simulink model "Aerotherme"  (R2019a)
settings: Solver=ode8  StartTime=0.0  StopTime=inf  FixedStep=0.1  RelTol=1e-3  EnableMultiTasking=on
values from neighbouring files (symbols this model uses):
  CorInt = tf(1 , [1 0])    [TP6.m]
  CorPD = tf([Td 1] , 1)*Kp    [TP6.m]
libraries: raspberrypilib x2, cstblocks x1
settings Model: SimulationMode=external  Creator=dorleans  LastModifiedBy=fereka231
settings SolverCC: PositivePriorityOrder=on
settings DataIOCC: ReturnWorkspaceOutputs=off
settings OptimizationCC: PassReuseOutputArgsAs=Individual arguments  MaxStackSize=64
settings DebuggingCC: ParameterPrecisionLossMsg=none  ParameterTunabilityLossMsg=error  SFUnexpectedBacktrackingDiag=warning  SFNoUnconditionalDefaultTransitionDiag=warning  ArithmeticOperatorsInVariantConditions=warning
settings HardwareCC: ProdBitPerPointer=32  ProdBitPerSizeT=32  ProdBitPerPtrDiffT=32  ProdLargestAtomicInteger=Long  ProdLargestAtomicFloat=Double  ProdWordSize=32  ProdHWDeviceType=ARM Compatible->ARM Cortex
settings ModelReferenceCC: PropagateSignalLabelsOutOfModel=off
settings SFSimCC: SimUseLocalCustomCode=off  MATLABDynamicMemAlloc=off
settings RTWCC: SystemTargetFile=ert.tlc  HardwareBoard=Raspberry Pi  TLCOptions="-aInlineSetEventsForThisBaseRateFcn=TLC_FALSE -aSuppressMultiTaskScheduler=TLC_FALSE  -aRateBasedStepFcn=0"  TemplateMakefile=ert_default_tmf  GenerateReport=on  RTWUseLocalCustomCode=off  Toolchain=GNU GCC Raspberry Pi  IncludeHyperlinkInReport=on  LaunchReport=on  GenerateTraceInfo=on  GenerateTraceReport=on  GenerateTraceReportSl=on  GenerateTraceReportSf=on  GenerateTraceReportEml=on
settings CodeAppCC: ForceParamTrailComments=on  IgnoreCustomStorageClasses=off  OperatorAnnotations=on  SimulinkDataObjDesc=on  SFDataObjDesc=on  MATLABFcnDesc=on  InsertBlockDesc=on  StateflowObjectComments=on  MATLABSourceComments=on
settings ERTTargetCC: SupportContinuousTime=on  SupportVariableSizeSignals=on

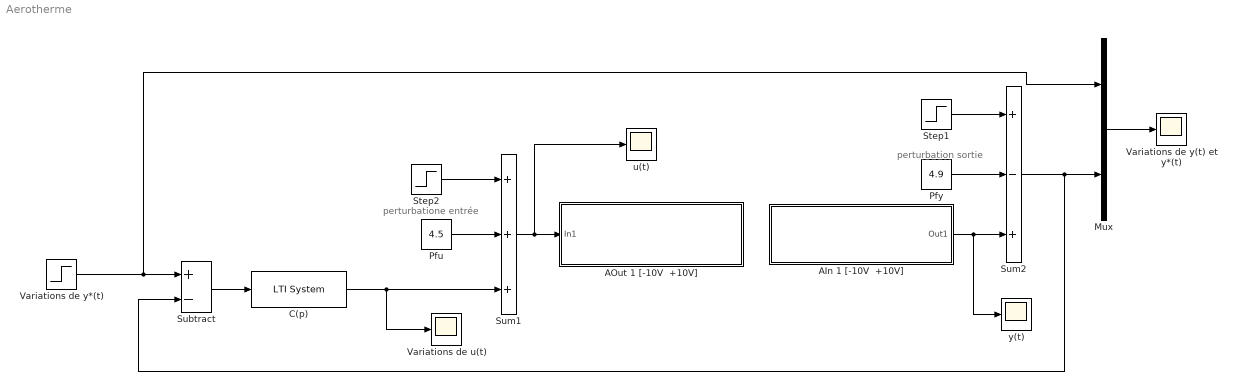
== system Aerotherme ==
  note: perturbatione entrée
  note: perturbation sortie
  AIn 1 [-10V  +10V] : Subsystem
      settings: OpenFcn=errordlg('Réalisé par Ph. Dorléans, H. Fleury','ESIX - UCBN')
      mask Display:
      | color('white');
      | plot([100,100,100,100],[100,100,100,100]);
      | plot([0,0,0,0],[0,0,0,0]);
      | color('blue');
      | text(99, 92, 'RASPBERRYPI', 'horizontalAlignment', 'right');
      | color('black');
      | text(50,60,'\fontsize{12}\bfAcquisition voie 1','texmode','on','horizontalAlignment','center','verticalAlignment','middle');
      | text(50,40,'\fontsize{10}\bfSPI Bus','texmode','on','horizontalAlignment','center','verticalAlignment','middle');
      | text(50,15,'Master Receiver SPI0 CE0' ,'horizontalAlignment', 'center');
  AOut 1 [-10V  +10V] : Subsystem
      settings: OpenFcn=errordlg('Réalisé par Ph. Dorléans, H. Fleury','ESIX - UCBN')
      mask Display:
      | color('white');
      | plot([100,100,100,100],[100,100,100,100]);
      | plot([0,0,0,0],[0,0,0,0]);
      | color('blue');
      | text(99, 92, 'RASPBERRYPI', 'horizontalAlignment', 'right');
      | color('black');
      | text(50,60,'\fontsize{12}\bfSortie analogique voie 1','texmode','on','horizontalAlignment','center','verticalAlignment','middle');
      | text(50,40,'\fontsize{10}\bfSPI Bus','texmode','on','horizontalAlignment','center','verticalAlignment','middle');
      | text(50,15,'Master Transfer SPI0 CE1' ,'horizontalAlignment', 'center');
  C(p) : cstblocks/LTI System  sys=CorInt*CorPD  IC=[]
  Mux : Mux  Inputs=2
  Pfu : Constant  Value=4.5
  Pfy : Constant  Value=4.9
  Step1 : Step  Time=0  After=0  SampleTime=0
  Step2 : Step  Time=0  SampleTime=0
  Subtract : Sum  Inputs=+-
  Sum1 : Sum  Inputs=+++  SaturateOnIntegerOverflow=on  InputSameDT=on  OutDataTypeStr=Inherit: Same as first input
  Sum2 : Sum  Inputs=+-+  SaturateOnIntegerOverflow=on  InputSameDT=on  OutDataTypeStr=Inherit: Same as first input
  Variations de u(t) : Scope
  Variations de y(t) et y*(t) : Scope
  Variations de y*(t) : Step  Time=0  SampleTime=0.1
  u(t) : Scope
  y(t) : Scope
  wires:
  Variations de y*(t)/1 -> Mux/1, Subtract/1
  Sum1/1 -> u(t)/1, AOut 1 [-10V  +10V]/1(In1)
  Subtract/1 -> C(p)/1
  C(p)/1 -> Variations de u(t)/1, Sum1/3
  AIn 1 [-10V  +10V]/1(Out1) -> y(t)/1, Sum2/3
  Sum2/1 -> Subtract/2, Mux/2
  Mux/1 -> Variations de y(t) et y*(t)/1
  Step2/1 -> Sum1/1
  Pfu/1 -> Sum1/2
  Step1/1 -> Sum2/1
  Pfy/1 -> Sum2/2

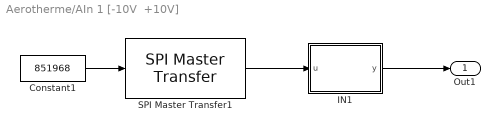
== system Aerotherme/AIn 1 [-10V  +10V] ==
  Constant1 : Constant  Value=851968  OutDataTypeStr=uint32  SampleTime=0.1
  IN1 : MATLAB Function  TreatAsAtomicUnit=on
  SPI Master Transfer1 : raspberrypilib/SPI Master Transfer  BoardProperty=Pi 3 Model B  SPIModule=uint32(0)  Mode=Master  BusSpeed=1000000  Pin=SPI0_CE0  FirstBitToTransfer=Most significant bit (MSB)  ClockMode=0  BlockFunction=Transfer  RegisterAddress=0  OutputDataType=int8  OutputDataLength=1
      settings: SourceProductName=Simulink Support Package for Raspberry Pi Hardware  SourceProductBaseCode=RASPPI
  Out1 : Outport
  wires:
  SPI Master Transfer1/1 -> IN1/1(u)
  Constant1/1 -> SPI Master Transfer1/1
  IN1/1(y) -> Out1/1

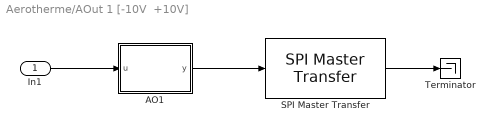
== system Aerotherme/AOut 1 [-10V  +10V] ==
  In1 : Inport
  AO1 : MATLAB Function  TreatAsAtomicUnit=on
  SPI Master Transfer : raspberrypilib/SPI Master Transfer  BoardProperty=Pi 3 Model B  SPIModule=uint32(0)  Mode=Master  BusSpeed=1000000  Pin=SPI0_CE1  FirstBitToTransfer=Most significant bit (MSB)  ClockMode=0  BlockFunction=Transfer  RegisterAddress=0  OutputDataType=int8  OutputDataLength=1
      settings: SourceProductName=Simulink Support Package for Raspberry Pi Hardware  SourceProductBaseCode=RASPPI
  Terminator : Terminator
  wires:
  SPI Master Transfer/1 -> Terminator/1
  AO1/1(y) -> SPI Master Transfer/1
  In1/1 -> AO1/1(u)

== matlab function Aerotherme/AIn 1 [-10V  +10V]/IN1 ==
  data: u input; y output
function y = fcn(u)

Vref = 3300;
offset = Vref/2;
coef = 10/offset

lecture = uint32(u)/8.0;

% masque = uint32(hex2dec('00000FFF'));   % pour assurer les 4 MSB à zéro
% lecture = bitand(lecture, masque); 

volts = lecture * Vref / 4095.0; 
volts = double(volts);
volts = (volts - offset) * coef;

y = volts;

== matlab function Aerotherme/AOut 1 [-10V  +10V]/AO1 ==
  data: u input; y output
function y = fcn(u)
% Envoi d'une tension comprise entre -10V et +10V
Vref = 4.096;

offset = 10;
coef = offset*2/3.3;
u = (u + offset) / coef; 

if (u > Vref) u = Vref;
end
if (u < 0)  u = 0;
end

nbr = ceil(u * 4095/Vref);      % convertisseur 12 bits  ->  2^12 - 1
                                % Arrondi à l'entier le + proche
nbr = uint16(nbr);              % Entier 16 bits non signé

masque = uint16(hex2dec('0FFF'));   % pour assurer les 4 MSB à zéro
resultat = bitand(nbr, masque); 


% bit 15 : 0 -> DAC A      1 -> DAC B
% bit 14 : 0 non utilisé
% bit 13 : 0 -> 2 Vref     1 -> Vref
% bit 12 : 1 active la conversion

masque = uint16(hex2dec('1000'));   % Positionner le bit 12 à 1 uniquement
resultat = bitor(resultat, masque); 
dec2hex(resultat);

y = resultat;
